simulink library "ddc_ufc_lib"  (R2024a)
settings: Solver=VariableStepAuto  StartTime=0.0  StopTime=10.0  RelTol=1e-3
settings Model: Creator=armangb1  LastModifiedBy=armangb1

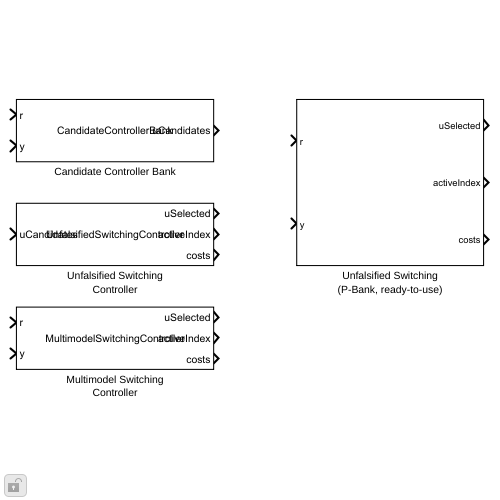
[thumbnail: Simulink's stored preview of the top-level diagram]
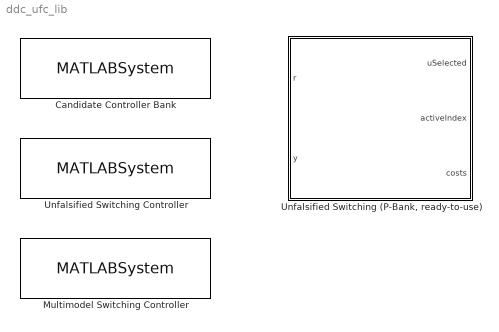
== system ddc_ufc_lib ==
  Candidate Controller Bank : MATLABSystem  System=ddc.ufc.CandidateControllerBank  Gains=[0.5;1;2]  SimulateUsing=Code generation
      mask Type: ddc.ufc.CandidateControllerBank
      mask Display:
      | disp('CandidateControllerBank');
      | port_label('input',1,'r');
      | port_label('input',2,'y');
      | port_label('output',1,'uCandidates');
  Multimodel Switching Controller : MATLABSystem  System=ddc.ufc.MultimodelSwitchingController  KpGains=[0.5;1;2]  KiGains=[0.1;0.2;0.5]  SampleTime=0.01  ForgettingFactor=0.95  HysteresisMargin=0.001  MinDwellSteps=5  ResetCostOnSwitch=on  SimulateUsing=Code generation
      mask Type: ddc.ufc.MultimodelSwitchingController
      mask Display:
      | disp('MultimodelSwitchingController');
      | port_label('input',1,'r');
      | port_label('input',2,'y');
      | port_label('output',1,'uSelected');
      | port_label('output',2,'activeIndex');
      | port_label('output',3,'costs');
  "Unfalsified Switching (P-Bank, ready-to-use)" : Subsystem  mask(Unfalsified Switching (P-Bank)){Gains=[0.5; 1; 2]}
      mask prompts: Gains "Candidate gains"
      mask help: Ready-to-use unfalsified adaptive switching control block: a bank of proportional candidate controllers plus the cost-based switching logic, pre-wired. Set Gains to the vector of candidate proportional gains.
  Unfalsified Switching Controller : MATLABSystem  System=ddc.ufc.UnfalsifiedSwitchingController  Gains=[0.5;1;2]  ForgettingFactor=0.95  HysteresisMargin=0.001  MinDwellSteps=5  ResetCostOnSwitch=on  SimulateUsing=Code generation
      mask Type: ddc.ufc.UnfalsifiedSwitchingController
      mask Display:
      | disp('UnfalsifiedSwitchingController');
      | port_label('input',1,'uCandidates');
      | port_label('output',1,'uSelected');
      | port_label('output',2,'activeIndex');
      | port_label('output',3,'costs');

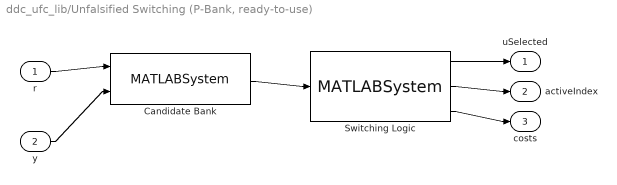
== system ddc_ufc_lib/Unfalsified Switching (P-Bank, ready-to-use) ==
  r : Inport
  y : Inport  Port=2
  Candidate Bank : MATLABSystem  System=ddc.ufc.CandidateControllerBank  Gains=Gains  SimulateUsing=Code generation
      mask Type: ddc.ufc.CandidateControllerBank
      mask Display:
      | disp('CandidateControllerBank');
      | port_label('input',1,'r');
      | port_label('input',2,'y');
      | port_label('output',1,'uCandidates');
  Switching Logic : MATLABSystem  System=ddc.ufc.UnfalsifiedSwitchingController  Gains=Gains  ForgettingFactor=0.95  HysteresisMargin=0.001  MinDwellSteps=5  ResetCostOnSwitch=on  SimulateUsing=Code generation
      mask Type: ddc.ufc.UnfalsifiedSwitchingController
      mask Display:
      | disp('UnfalsifiedSwitchingController');
      | port_label('input',1,'uCandidates');
      | port_label('output',1,'uSelected');
      | port_label('output',2,'activeIndex');
      | port_label('output',3,'costs');
  uSelected : Outport
  activeIndex : Outport  Port=2
  costs : Outport  Port=3
  wires:
  r/1 -> Candidate Bank/1
  y/1 -> Candidate Bank/2
  Candidate Bank/1 -> Switching Logic/1
  Switching Logic/1 -> uSelected/1
  Switching Logic/2 -> activeIndex/1
  Switching Logic/3 -> costs/1
